simulink model "ODE_neurospora_model_leloup_za_sliko"  (R2015a)
settings: Solver=ode4  StartTime=0.0  StopTime=72  FixedStep=0.000278  RelTol=1e-3
values from neighbouring files (symbols this model uses):
  k_1 = 0.5    [ALL_neurospora_init.m]    (also in FUZZY_deg_neurospora_init.m; FUZZY_tsc_neurospora_init.m; FUZZY_tsc_tsl_neurospora_init.m; FUZZY_tsl_neurospora_init.m)
  k_2 = 0.6    [ALL_neurospora_init.m]    (also in FUZZY_deg_neurospora_init.m; FUZZY_tsc_neurospora_init.m; FUZZY_tsc_tsl_neurospora_init.m; FUZZY_tsl_neurospora_init.m)
  K_d = 0.13    [ALL_neurospora_init.m]    (also in FUZZY_deg_neurospora_init.m; FUZZY_tsc_neurospora_init.m; FUZZY_tsc_tsl_neurospora_init.m; FUZZY_tsl_neurospora_init.m)
  K_I = 1    [ALL_neurospora_init.m]    (also in FUZZY_deg_neurospora_init.m; FUZZY_tsc_neurospora_init.m; FUZZY_tsc_tsl_neurospora_init.m; FUZZY_tsl_neurospora_init.m)
  K_m = 0.5    [ALL_neurospora_init.m]    (also in FUZZY_deg_neurospora_init.m; FUZZY_tsc_neurospora_init.m; FUZZY_tsc_tsl_neurospora_init.m; FUZZY_tsl_neurospora_init.m)
  k_s = 0.5    [ALL_neurospora_init.m]    (also in FUZZY_deg_neurospora_init.m; FUZZY_tsc_neurospora_init.m; FUZZY_tsc_tsl_neurospora_init.m; FUZZY_tsl_neurospora_init.m)
  n = 4    [ALL_neurospora_init.m]    (also in FUZZY_deg_neurospora_init.m; FUZZY_tsc_neurospora_init.m; FUZZY_tsc_tsl_neurospora_init.m; FUZZY_tsl_neurospora_init.m)
  v_d = 1.4    [ALL_neurospora_init.m]    (also in FUZZY_deg_neurospora_init.m; FUZZY_tsc_neurospora_init.m; FUZZY_tsc_tsl_neurospora_init.m; FUZZY_tsl_neurospora_init.m)
  v_m = 0.505    [ALL_neurospora_init.m]    (also in FUZZY_deg_neurospora_init.m; FUZZY_tsc_neurospora_init.m; FUZZY_tsc_tsl_neurospora_init.m; FUZZY_tsl_neurospora_init.m)
  v_s = 1.6    [ALL_neurospora_init.m]    (also in FUZZY_deg_neurospora_init.m; FUZZY_tsc_neurospora_init.m; FUZZY_tsc_tsl_neurospora_init.m; FUZZY_tsl_neurospora_init.m)
settings Model: Creator=jureb  LastModifiedBy=jureb

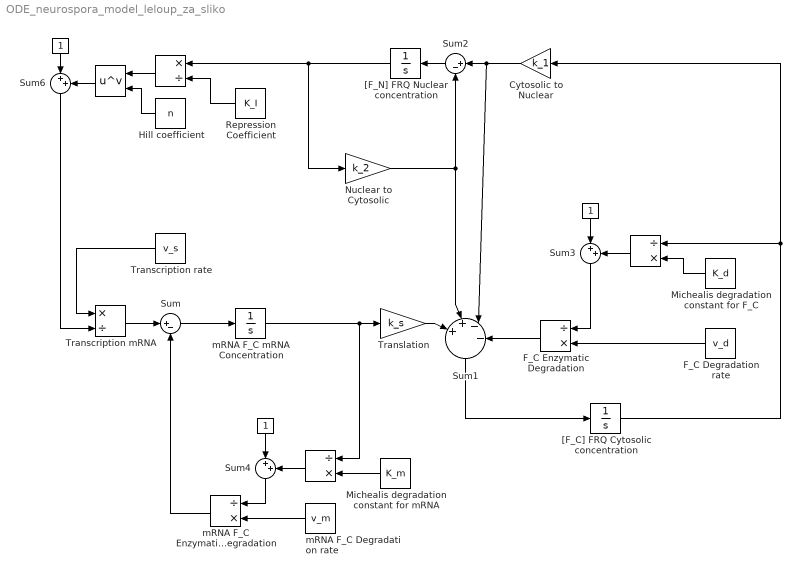
== system ODE_neurospora_model_leloup_za_sliko ==
  " " : Math  Operator=pow  SaturateOnIntegerOverflow=on
  " " : Product  Inputs=/*
  " " : Product  Inputs=*/
  "          " : Constant
  " " : Constant
  " " : Constant
  " " : Product  Inputs=/*
  Cytosolic to Nuclear : Gain  Gain=k_1
  F_C Degradation rate : Constant  Value=v_d
  F_C Enzymatic Degradation : Product  Inputs=/*
  Hill coefficient : Constant  Value=n
  Michealis degradation constant for F_C : Constant  Value=K_d
  Michealis degradation constant for mRNA : Constant  Value=K_m
  Nuclear to Cytosolic : Gain  Gain=k_2
  Repression Coefficient : Constant  Value=K_I
  Sum : Sum  Inputs=|+-
  Sum1 : Sum  Inputs=|+|+|-|-
  Sum2 : Sum  Inputs=|+-
  Sum3 : Sum  Inputs=|++
  Sum4 : Sum  Inputs=|++
  Sum6 : Sum  Inputs=|++
  Transcription mRNA : Product  Inputs=*/
  Transcription rate : Constant  Value=v_s
  Translation : Gain  Gain=k_s
  "[F_C] FRQ Cytosolic concentration " : Integrator  InitialCondition=1
  "[F_N] FRQ Nuclear concentration" : Integrator  InitialCondition=1
  mRNA F_C Degradation rate : Constant  Value=v_m
  mRNA F_C Enzymatic Degradation : Product  Inputs=/*
  mRNA F_C mRNA Concentration : Integrator  InitialCondition=1
  wires:
  Sum6/1 -> Transcription mRNA/2
  "          "/1 -> Sum6/1
  Transcription mRNA/1 -> Sum/1
  " "/1 -> Sum6/2
  Hill coefficient/1 -> " "/2
  Sum/1 -> mRNA F_C mRNA Concentration/1
  " "/1 -> " "/1
  mRNA F_C mRNA Concentration/1 -> " "/1, Translation/1
  mRNA F_C Enzymatic Degradation/1 -> Sum/2
  "[F_N] FRQ Nuclear concentration"/1 -> " "/1, Nuclear to Cytosolic/1
  Repression Coefficient/1 -> " "/2
  Sum1/1 -> "[F_C] FRQ Cytosolic concentration "/1
  Cytosolic to Nuclear/1 -> Sum1/3, Sum2/1
  Sum2/1 -> "[F_N] FRQ Nuclear concentration"/1
  Nuclear to Cytosolic/1 -> Sum1/2, Sum2/2
  mRNA F_C Degradation rate/1 -> mRNA F_C Enzymatic Degradation/2
  " "/1 -> Sum4/1
  " "/1 -> Sum4/2
  Michealis degradation constant for mRNA/1 -> " "/2
  Sum4/1 -> mRNA F_C Enzymatic Degradation/1
  "[F_C] FRQ Cytosolic concentration "/1 -> Cytosolic to Nuclear/1, " "/1
  F_C Enzymatic Degradation/1 -> Sum1/4
  F_C Degradation rate/1 -> F_C Enzymatic Degradation/2
  " "/1 -> Sum3/1
  " "/1 -> Sum3/2
  Michealis degradation constant for F_C/1 -> " "/2
  Sum3/1 -> F_C Enzymatic Degradation/1
  Translation/1 -> Sum1/1
  Transcription rate/1 -> Transcription mRNA/1
